simulink model "gain_test_Kuuvect"  (Simulink 7.2)
settings: Solver=ode45  StartTime=0.0  StopTime=10.0  RelTol=1e-3
settings Model: Creator=arnaud  LastModifiedBy=arnaud
settings DataIOCC: SaveFormat=Structure

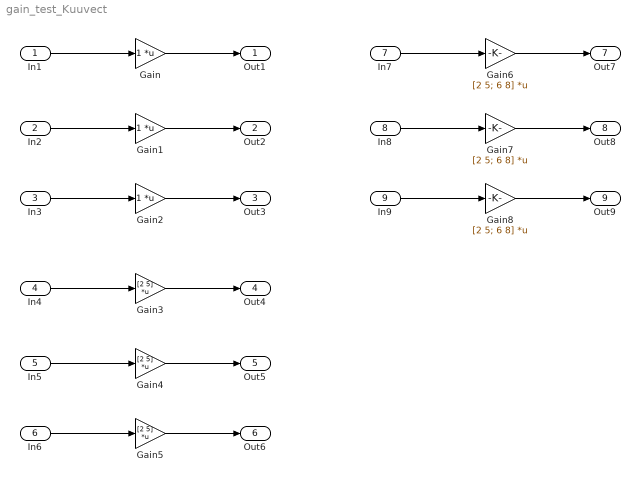
== system gain_test_Kuuvect ==
  In1 : Inport  DataType=double  OutDataType=sfix(16)  OutScaling=2^0  OutDataTypeStr=double
  In2 : Inport  Port=2  PortDimensions=1  DataType=int8  OutDataType=sfix(16)  OutScaling=2^0  OutDataTypeStr=int8
  In3 : Inport  Port=3  PortDimensions=1  DataType=boolean  OutDataType=sfix(16)  OutScaling=2^0  OutDataTypeStr=boolean
  In4 : Inport  Port=4  PortDimensions=2  DataType=double  OutDataType=sfix(16)  OutScaling=2^0  OutDataTypeStr=double
  In5 : Inport  Port=5  DataType=int8  OutDataType=sfix(16)  OutScaling=2^0  OutDataTypeStr=int8
  In6 : Inport  Port=6  DataType=boolean  OutDataType=sfix(16)  OutScaling=2^0  OutDataTypeStr=boolean
  In7 : Inport  Port=7  PortDimensions=[2 1]  DataType=double  OutDataType=sfix(16)  OutScaling=2^0  OutDataTypeStr=double
  In8 : Inport  Port=8  PortDimensions=[1 2]  DataType=int8  OutDataType=sfix(16)  OutScaling=2^0  OutDataTypeStr=int8
  In9 : Inport  Port=9  PortDimensions=[2 1]  DataType=boolean  OutDataType=sfix(16)  OutScaling=2^0  OutDataTypeStr=boolean
  Gain : Gain  Multiplication=Matrix(K*u) (u vector)  ParameterDataType=sfix(16)  ParameterScaling=2^0  OutDataType=sfix(16)  OutScaling=2^0
  Gain1 : Gain  Multiplication=Matrix(K*u) (u vector)  ParameterDataType=sfix(16)  ParameterScaling=2^0  OutDataType=sfix(16)  OutScaling=2^0
  Gain2 : Gain  Multiplication=Matrix(K*u) (u vector)  ParameterDataType=sfix(16)  ParameterScaling=2^0  OutDataType=sfix(16)  OutScaling=2^0
  Gain3 : Gain  Gain=[2 5]  Multiplication=Matrix(K*u) (u vector)  ParameterDataType=sfix(16)  ParameterScaling=2^0  OutDataType=sfix(16)  OutScaling=2^0
  Gain4 : Gain  Gain=[2 5]  Multiplication=Matrix(K*u) (u vector)  ParameterDataType=sfix(16)  ParameterScaling=2^0  OutDataType=sfix(16)  OutScaling=2^0
  Gain5 : Gain  Gain=[2 5]  Multiplication=Matrix(K*u) (u vector)  ParameterDataType=sfix(16)  ParameterScaling=2^0  OutDataType=sfix(16)  OutScaling=2^0
  Gain6 : Gain  Gain=[2 5; 6 8]  Multiplication=Matrix(K*u) (u vector)  ParameterDataType=sfix(16)  ParameterScaling=2^0  OutDataType=sfix(16)  OutScaling=2^0
  Gain7 : Gain  Gain=[2 5; 6 8]  Multiplication=Matrix(K*u) (u vector)  ParameterDataType=sfix(16)  ParameterScaling=2^0  OutDataType=sfix(16)  OutScaling=2^0
  Gain8 : Gain  Gain=[2 5; 6 8]  Multiplication=Matrix(K*u) (u vector)  ParameterDataType=sfix(16)  ParameterScaling=2^0  OutDataType=sfix(16)  OutScaling=2^0
  Out1 : Outport  OutDataType=sfix(16)  OutScaling=2^0
  Out2 : Outport  Port=2  OutDataType=sfix(16)  OutScaling=2^0
  Out3 : Outport  Port=3  OutDataType=sfix(16)  OutScaling=2^0
  Out4 : Outport  Port=4  OutDataType=sfix(16)  OutScaling=2^0
  Out5 : Outport  Port=5  OutDataType=sfix(16)  OutScaling=2^0
  Out6 : Outport  Port=6  OutDataType=sfix(16)  OutScaling=2^0
  Out7 : Outport  Port=7  OutDataType=sfix(16)  OutScaling=2^0
  Out8 : Outport  Port=8  OutDataType=sfix(16)  OutScaling=2^0
  Out9 : Outport  Port=9  OutDataType=sfix(16)  OutScaling=2^0
  wires:
  In1/1 -> Gain/1
  Gain/1 -> Out1/1
  In2/1 -> Gain1/1
  Gain1/1 -> Out2/1
  In3/1 -> Gain2/1
  Gain2/1 -> Out3/1
  In4/1 -> Gain3/1
  Gain3/1 -> Out4/1
  In5/1 -> Gain4/1
  Gain4/1 -> Out5/1
  In6/1 -> Gain5/1
  Gain5/1 -> Out6/1
  In7/1 -> Gain6/1
  Gain6/1 -> Out7/1
  In8/1 -> Gain7/1
  Gain7/1 -> Out8/1
  In9/1 -> Gain8/1
  Gain8/1 -> Out9/1
